simulink model "ex4"  (R2020a)
settings: Solver=VariableStepAuto  StartTime=0.0  StopTime=10.0  RelTol=1e-3
undefined symbols (not defined in the file): A, B, C, D
settings Model: Creator=EREN  LastModifiedBy=EREN

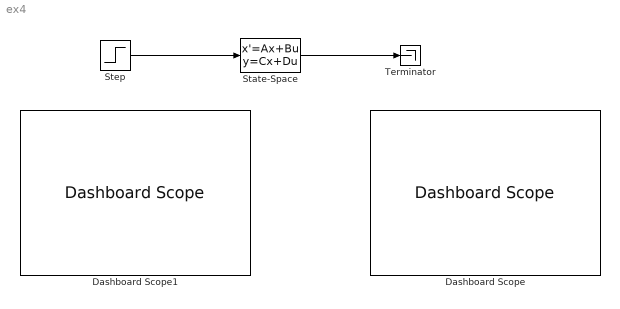
== system ex4 ==
  Dashboard Scope : DashboardScope
  Dashboard Scope1 : DashboardScope
  State-Space : StateSpace  A=A  B=B  C=C  D=D  InitialCondition=0
  Step : Step  Time=0  After=7  SampleTime=0
  Terminator : Terminator
  wires:
  State-Space/1 -> Terminator/1
  Step/1 -> State-Space/1
